simulink model "certasian_traj"  (R2020a)
settings: Solver=VariableStepAuto  StartTime=0.0  StopTime=10.0  RelTol=1e-3
libraries: dsppolyfun x3, simulink x3
settings Model: Creator=UNIST  LastModifiedBy=UNIST

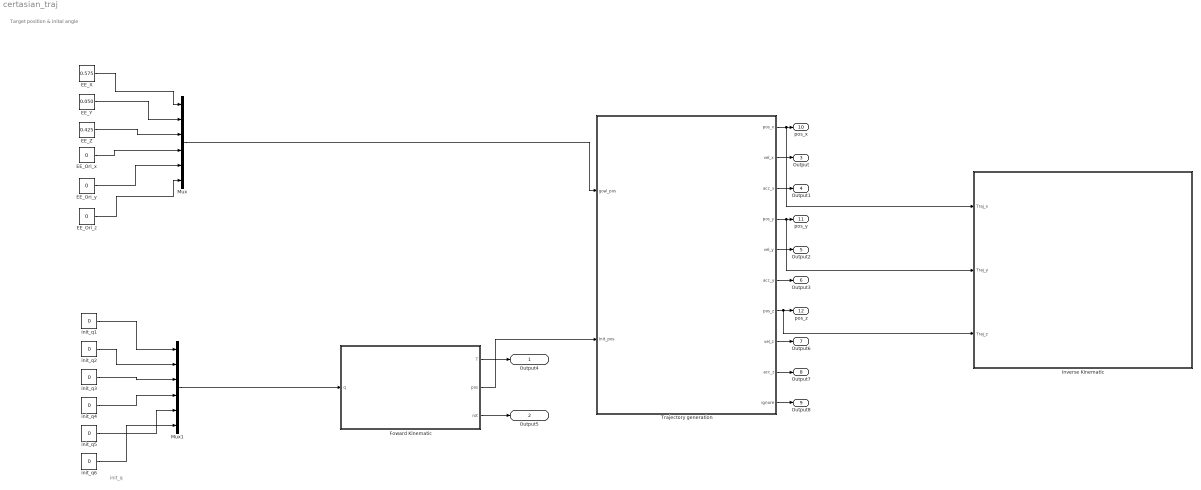
== system certasian_traj ==
  note: Target position & inital angle
  note: init_q
  EE_Ori_x : Constant  Value=0
  EE_Ori_y : Constant  Value=0
  EE_Ori_z : Constant  Value=0
  EE_X : Constant  Value=0.575
  EE_Y : Constant  Value=0.050
  EE_Z : Constant  Value=0.425
  Foward Kinematic : MATLAB Function  TreatAsAtomicUnit=on
  Inverse Kinematic : Subsystem
  Mux : Mux  Inputs=6
  Mux1 : Mux  Inputs=6
  Trajectory generation : Subsystem
  init_q{1..6} (6 alike) : Constant  Value=0
  Output4 : Outport
  Output5 : Outport  Port=2
  Output : Outport  Port=3
  Output1 : Outport  Port=4
  Output2 : Outport  Port=5
  Output3 : Outport  Port=6
  Output6 : Outport  Port=7
  Output7 : Outport  Port=8
  Output8 : Outport  Port=9
  pos_x : Outport  Port=10
  pos_y : Outport  Port=11
  pos_z : Outport  Port=12
  wires:
  EE_Y/1 -> Mux/2
  EE_Ori_x/1 -> Mux/4
  Mux/1 -> Trajectory generation/1(goal_pos)
  init_q6/1 -> Mux1/6
  init_q3/1 -> Mux1/3
  init_q5/1 -> Mux1/5
  EE_Ori_y/1 -> Mux/5
  EE_X/1 -> Mux/1
  init_q1/1 -> Mux1/1
  init_q4/1 -> Mux1/4
  EE_Ori_z/1 -> Mux/6
  init_q2/1 -> Mux1/2
  EE_Z/1 -> Mux/3
  Mux1/1 -> Foward Kinematic/1(q)
  Foward Kinematic/1(T) -> Output4/1
  Foward Kinematic/3(rot) -> Output5/1
  Trajectory generation/2(vel_x) -> Output/1
  Trajectory generation/3(acc_x) -> Output1/1
  Trajectory generation/5(vel_y) -> Output2/1
  Trajectory generation/6(acc_y) -> Output3/1
  Trajectory generation/8(vel_z) -> Output6/1
  Trajectory generation/9(acc_z) -> Output7/1
  Foward Kinematic/2(pos) -> Trajectory generation/2(Init_pos)
  Trajectory generation/10(ignore) -> Output8/1
  Trajectory generation/1(pos_x) -> pos_x/1, Inverse Kinematic/1(Traj_x)
  Trajectory generation/4(pos_y) -> Inverse Kinematic/2(Traj_y), pos_y/1
  Trajectory generation/7(pos_z) -> Inverse Kinematic/3(Traj_z), pos_z/1

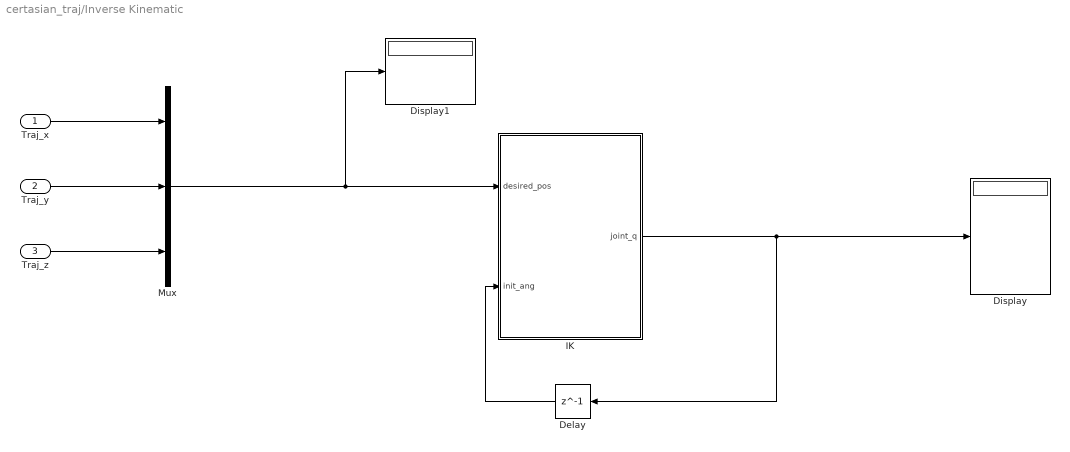
== system certasian_traj/Inverse Kinematic ==
  Traj_x : Inport
  Traj_y : Inport  Port=2
  Traj_z : Inport  Port=3
  Delay : Delay  DelayLength=1
  Display : Display
  Display1 : Display
  IK : MATLAB Function  TreatAsAtomicUnit=on
  Mux : Mux  Inputs=3
  wires:
  Traj_x/1 -> Mux/1
  Traj_y/1 -> Mux/2
  Traj_z/1 -> Mux/3
  Mux/1 -> Display1/1, IK/1(desired_pos)
  IK/1(joint_q) -> Delay/1, Display/1
  Delay/1 -> IK/2(init_ang)

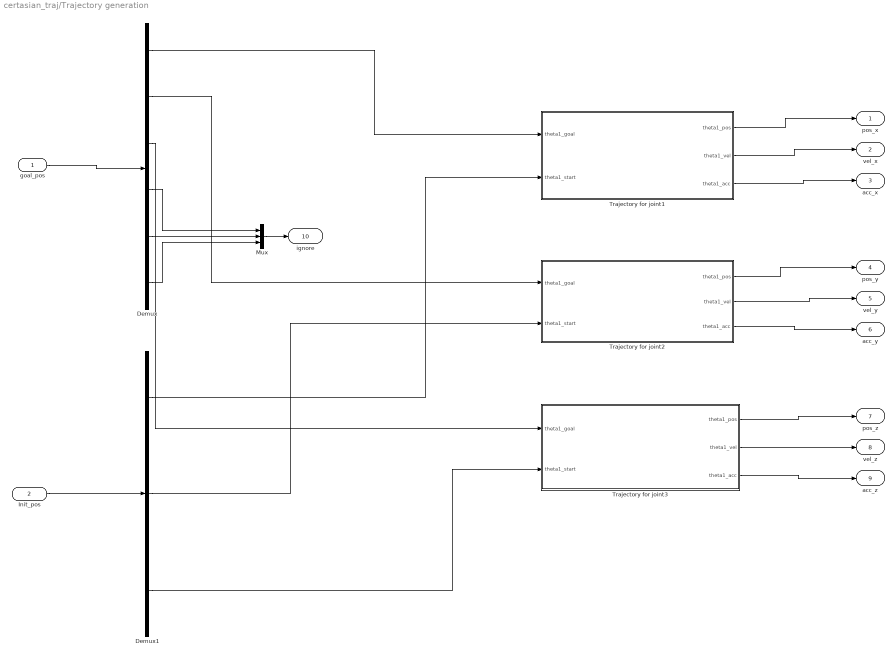
== system certasian_traj/Trajectory generation ==
  goal_pos : Inport
  Init_pos : Inport  Port=2
  Demux : Demux  Outputs=6
  Demux1 : Demux  Outputs=3
  Mux : Mux  Inputs=3
  Trajectory for joint1 : Subsystem
  Trajectory for joint2 : Subsystem
  Trajectory for joint3 : Subsystem
  pos_x : Outport
  vel_x : Outport  Port=2
  acc_x : Outport  Port=3
  pos_y : Outport  Port=4
  vel_y : Outport  Port=5
  acc_y : Outport  Port=6
  pos_z : Outport  Port=7
  vel_z : Outport  Port=8
  acc_z : Outport  Port=9
  ignore : Outport  Port=10
  wires:
  goal_pos/1 -> Demux/1
  Init_pos/1 -> Demux1/1
  Trajectory for joint1/1("theta1_pos ") -> pos_x/1
  Trajectory for joint1/2("theta1_vel ") -> vel_x/1
  Trajectory for joint2/1("theta1_pos ") -> pos_y/1
  Trajectory for joint2/3("theta1_acc ") -> acc_y/1
  Trajectory for joint1/3("theta1_acc ") -> acc_x/1
  Trajectory for joint3/1("theta1_pos ") -> pos_z/1
  Trajectory for joint3/3("theta1_acc ") -> acc_z/1
  Trajectory for joint3/2("theta1_vel ") -> vel_z/1
  Demux/4 -> Mux/1
  Demux/5 -> Mux/2
  Demux/6 -> Mux/3
  Mux/1 -> ignore/1
  Demux/1 -> Trajectory for joint1/1("theta1_goal ")
  Demux1/1 -> Trajectory for joint1/2("theta1_start ")
  Trajectory for joint2/2("theta1_vel ") -> vel_y/1
  Demux/2 -> Trajectory for joint2/1("theta1_goal ")
  Demux1/2 -> Trajectory for joint2/2("theta1_start ")
  Demux/3 -> Trajectory for joint3/1("theta1_goal ")
  Demux1/3 -> Trajectory for joint3/2("theta1_start ")

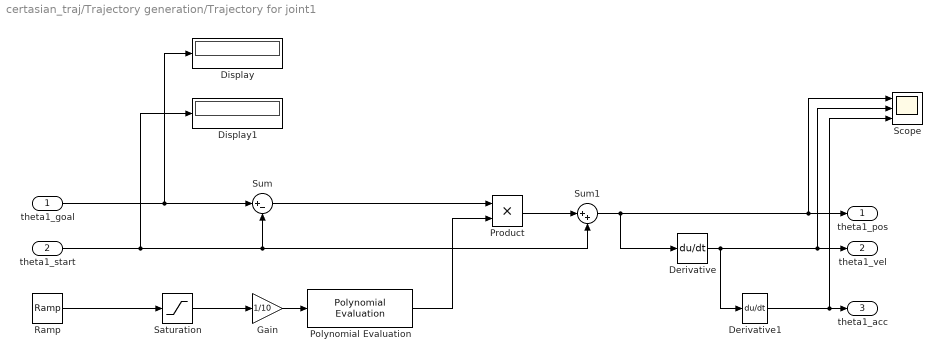
== system certasian_traj/Trajectory generation/Trajectory for joint1 ==
  "theta1_goal " : Inport
  "theta1_start " : Inport  Port=2
  Derivative : Derivative
  Derivative1 : Derivative
  Display : Display
  Display1 : Display
  Gain : Gain  Gain=1/10
  Polynomial Evaluation : dsppolyfun/Polynomial Evaluation  useConstCoeffs=on  constCoeffs=[6 -15 10 0 0 0]
      settings: SourceProductBaseCode=DS
  Product : Product
  Ramp : simulink/Sources/Ramp  slope=1  start=0  InitialOutput=0
  Saturation : Saturate  UpperLimit=10  LowerLimit=-10
  Scope : Scope  NumInputPorts=3
  Sum : Sum  Inputs=|+-
  Sum1 : Sum  Inputs=|++
  "theta1_pos " : Outport  VectorParamsAs1DForOutWhenUnconnected=off
  "theta1_vel " : Outport  Port=2  VectorParamsAs1DForOutWhenUnconnected=off
  "theta1_acc " : Outport  Port=3  VectorParamsAs1DForOutWhenUnconnected=off
  wires:
  "theta1_start "/1 -> Sum1/2, Sum/2, Display1/1
  Sum/1 -> Product/1
  "theta1_goal "/1 -> Display/1, Sum/1
  Sum1/1 -> Derivative/1, Scope/1, "theta1_pos "/1
  Derivative/1 -> Scope/2, "theta1_vel "/1, Derivative1/1
  Gain/1 -> Polynomial Evaluation/1
  Product/1 -> Sum1/1
  Polynomial Evaluation/1 -> Product/2
  Derivative1/1 -> Scope/3, "theta1_acc "/1
  Saturation/1 -> Gain/1
  Ramp/1 -> Saturation/1

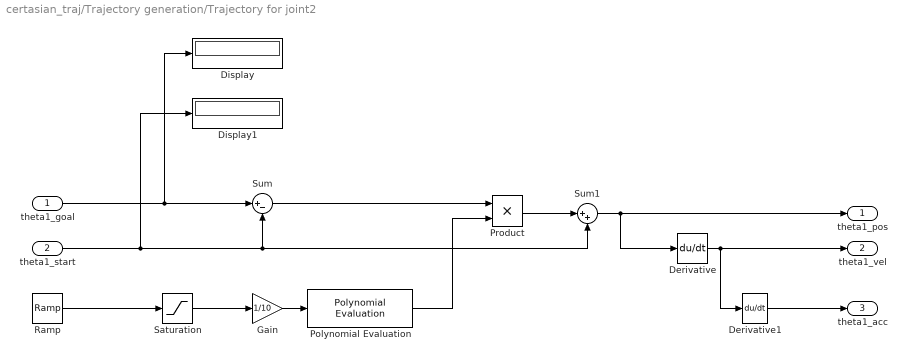
== system certasian_traj/Trajectory generation/Trajectory for joint2 ==
  "theta1_goal " : Inport
  "theta1_start " : Inport  Port=2
  Derivative : Derivative
  Derivative1 : Derivative
  Display : Display
  Display1 : Display
  Gain : Gain  Gain=1/10
  Polynomial Evaluation : dsppolyfun/Polynomial Evaluation  useConstCoeffs=on  constCoeffs=[6 -15 10 0 0 0]
      settings: SourceProductBaseCode=DS
  Product : Product
  Ramp : simulink/Sources/Ramp  slope=1  start=0  InitialOutput=0
  Saturation : Saturate  UpperLimit=10  LowerLimit=-10
  Sum : Sum  Inputs=|+-
  Sum1 : Sum  Inputs=|++
  "theta1_pos " : Outport  VectorParamsAs1DForOutWhenUnconnected=off
  "theta1_vel " : Outport  Port=2  VectorParamsAs1DForOutWhenUnconnected=off
  "theta1_acc " : Outport  Port=3  VectorParamsAs1DForOutWhenUnconnected=off
  wires:
  "theta1_start "/1 -> Sum1/2, Sum/2, Display1/1
  Sum/1 -> Product/1
  "theta1_goal "/1 -> Display/1, Sum/1
  Sum1/1 -> Derivative/1, "theta1_pos "/1
  Derivative/1 -> "theta1_vel "/1, Derivative1/1
  Gain/1 -> Polynomial Evaluation/1
  Product/1 -> Sum1/1
  Polynomial Evaluation/1 -> Product/2
  Derivative1/1 -> "theta1_acc "/1
  Saturation/1 -> Gain/1
  Ramp/1 -> Saturation/1

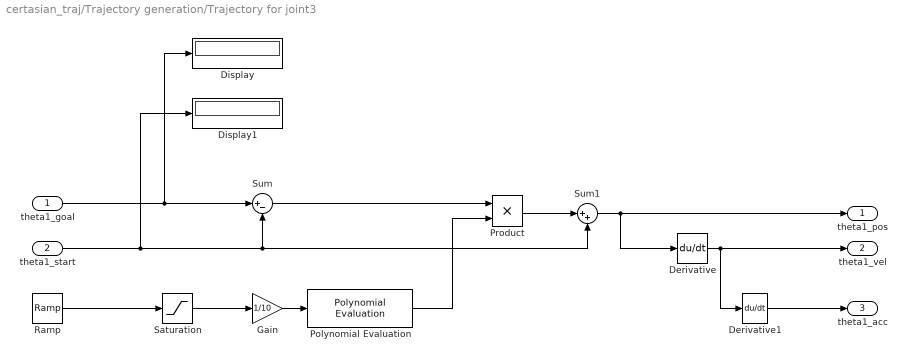
== system certasian_traj/Trajectory generation/Trajectory for joint3 ==
  "theta1_goal " : Inport
  "theta1_start " : Inport  Port=2
  Derivative : Derivative
  Derivative1 : Derivative
  Display : Display
  Display1 : Display
  Gain : Gain  Gain=1/10
  Polynomial Evaluation : dsppolyfun/Polynomial Evaluation  useConstCoeffs=on  constCoeffs=[6 -15 10 0 0 0]
      settings: SourceProductBaseCode=DS
  Product : Product
  Ramp : simulink/Sources/Ramp  slope=1  start=0  InitialOutput=0
  Saturation : Saturate  UpperLimit=10  LowerLimit=-10
  Sum : Sum  Inputs=|+-
  Sum1 : Sum  Inputs=|++
  "theta1_pos " : Outport  VectorParamsAs1DForOutWhenUnconnected=off
  "theta1_vel " : Outport  Port=2  VectorParamsAs1DForOutWhenUnconnected=off
  "theta1_acc " : Outport  Port=3  VectorParamsAs1DForOutWhenUnconnected=off
  wires:
  "theta1_start "/1 -> Sum1/2, Sum/2, Display1/1
  Sum/1 -> Product/1
  "theta1_goal "/1 -> Display/1, Sum/1
  Sum1/1 -> Derivative/1, "theta1_pos "/1
  Derivative/1 -> "theta1_vel "/1, Derivative1/1
  Gain/1 -> Polynomial Evaluation/1
  Product/1 -> Sum1/1
  Polynomial Evaluation/1 -> Product/2
  Derivative1/1 -> "theta1_acc "/1
  Saturation/1 -> Gain/1
  Ramp/1 -> Saturation/1

== matlab function certasian_traj/Foward Kinematic ==
  data: q input; T output; pos output; rot output
function [T,pos,rot] = FK(q)

theta1=q(1);  d1=0;   a1=0.050;  alpha1=-90; %parameter link1
theta2=q(2);  d2=0.050;   a2=0.425;  alpha2=0; %parameter link2
theta3=q(3);  d3=0;  a3=0;  alpha3=90; %parameter link3
theta4=q(4);  d4=0.425;   a4=0;  alpha4=-90; %parameter link4
theta5=q(5);  d5=0; a5=0;  alpha5=90; %parameter link5
theta6=q(6);  d6=0.100; a6=0;  alpha6=0; %parameter link6
offset2 = -90;
offset3 = 90;
T01=[cosd(theta1) -cosd(alpha1)*sind(theta1) sind(alpha1)*sind(theta1) a1*cosd(theta1);
    sind(theta1) cosd(alpha1)*cosd(theta1)  -sind(alpha1)*cosd(theta1) a1*sind(theta1);
    0,sind(alpha1),cosd(alpha1),d1;
    0,0,0,1];
T12=[cosd(theta2+offset2) -cosd(alpha2)*sind(theta2+offset2) sind(alpha2)*sind(theta2+offset2) a2*cosd(theta2+offset2);
    sind(theta2+offset2) cosd(alpha2)*cosd(theta2+offset2)  -sind(alpha2)*cosd(theta2+offset2) a2*sind(theta2+offset2);
    0,sind(alpha2),cosd(alpha2),d2;
    0,0,0,1];
T23=[cosd(theta3+offset3) -cosd(alpha3)*sind(theta3+offset3) sind(alpha3)*sind(theta3+offset3) a3*cosd(theta3+offset3);
    sind(theta3+offset3) cosd(alpha3)*cosd(theta3+offset3)  -sind(alpha3)*cosd(theta3+offset3) a3*sind(theta3+offset3);
    0,sind(alpha3),cosd(alpha3),d3;
    0,0,0,1];
T34=[cosd(theta4) -cosd(alpha4)*sind(theta4) sind(alpha4)*sind(theta4) a4*cosd(theta4);
     sind(theta4) cosd(alpha4)*cosd(theta4)  -sind(alpha4)*cosd(theta4) a4*sind(theta4);
     0,sind(alpha4),cosd(alpha4),d4;
     0,0,0,1];
T45=[cosd(theta5) -cosd(alpha5)*sind(theta5) sind(alpha5)*sind(theta5) a5*cosd(theta5);
     sind(theta5) cosd(alpha5)*cosd(theta5)  -sind(alpha5)*cosd(theta5) a5*sind(theta5);
     0,sind(alpha5),cosd(alpha5),d5;
     0,0,0,1];
T56=[cosd(theta6) -cosd(alpha6)*sind(theta6) sind(alpha6)*sind(theta6) a6*cosd(theta6);
     sind(theta6) cosd(alpha6)*cosd(theta6)  -sind(alpha6)*cosd(theta6) a6*sind(theta6);
     0,sind(alpha6),cosd(alpha6),d6;
     0,0,0,1];
T01;
T02 = T01*T12;
T03 = T01*T12*T23;
T04 = T01*T12*T23*T34;
T05 = T01*T12*T23*T34*T45;
T06 = T01*T12*T23*T34*T45*T56;
P6=T06(1:3,4);
R = [T06(1:3,1) T06(1:3,2) T06(1:3,3)]; 
T = T06;
pos = P6;
rot = R;

== matlab function certasian_traj/Inverse Kinematic/IK ==
  data: desired_pos input; joint_q output; init_ang input
function joint_q = IK(desired_pos, init_ang)

theta1=init_ang(1);  d1=0;   a1=0.050;  alpha1=-90; %parameter link1
theta2=init_ang(2);  d2=0.050;   a2=0.425;  alpha2=0; %parameter link2
theta3=init_ang(3);  d3=0;  a3=0;  alpha3=90; %parameter link3
theta4=init_ang(4);  d4=0.425;   a4=0;  alpha4=-90; %parameter link4
theta5=init_ang(5);  d5=0; a5=0;  alpha5=90; %parameter link5
theta6=init_ang(6);  d6=0.100; a6=0;  alpha6=0; %parameter link6

offset2 = -90;
offset3 = 90;

T01=[cosd(theta1) -cosd(alpha1)*sind(theta1) sind(alpha1)*sind(theta1) a1*cosd(theta1);
sind(theta1) cosd(alpha1)*cosd(theta1)  -sind(alpha1)*cosd(theta1) a1*sind(theta1);
0,sind(alpha1),cosd(alpha1),d1;
0,0,0,1];
T12=[cosd(theta2+offset2) -cosd(alpha2)*sind(theta2+offset2) sind(alpha2)*sind(theta2+offset2) a2*cosd(theta2+offset2);
sind(theta2+offset2) cosd(alpha2)*cosd(theta2+offset2)  -sind(alpha2)*cosd(theta2+offset2) a2*sind(theta2+offset2);
0,sind(alpha2),cosd(alpha2),d2;
0,0,0,1];
T23=[cosd(theta3+offset3) -cosd(alpha3)*sind(theta3+offset3) sind(alpha3)*sind(theta3+offset3) a3*cosd(theta3+offset3);
sind(theta3+offset3) cosd(alpha3)*cosd(theta3+offset3)  -sind(alpha3)*cosd(theta3+offset3) a3*sind(theta3+offset3);
0,sind(alpha3),cosd(alpha3),d3;
0,0,0,1];
T34=[cosd(theta4) -cosd(alpha4)*sind(theta4) sind(alpha4)*sind(theta4) a4*cosd(theta4);
 sind(theta4) cosd(alpha4)*cosd(theta4)  -sind(alpha4)*cosd(theta4) a4*sind(theta4);
 0,sind(alpha4),cosd(alpha4),d4;
 0,0,0,1];
T45=[cosd(theta5) -cosd(alpha5)*sind(theta5) sind(alpha5)*sind(theta5) a5*cosd(theta5);
 sind(theta5) cosd(alpha5)*cosd(theta5)  -sind(alpha5)*cosd(theta5) a5*sind(theta5);
 0,sind(alpha5),cosd(alpha5),d5;
 0,0,0,1];
T56=[cosd(theta6) -cosd(alpha6)*sind(theta6) sind(alpha6)*sind(theta6) a6*cosd(theta6);
 sind(theta6) cosd(alpha6)*cosd(theta6)  -sind(alpha6)*cosd(theta6) a6*sind(theta6);
 0,sind(alpha6),cosd(alpha6),d6;
 0,0,0,1];
T01;
T02 = T01*T12;
T03 = T01*T12*T23;
T04 = T01*T12*T23*T34;
T05 = T01*T12*T23*T34*T45;
T06 = T01*T12*T23*T34*T45*T56;
P6=T06(1:3,4);
iteration = 0;
b = 0 ;
deltatheta1=0;deltatheta2=0; deltatheta3=0; %theta1,2,3 velocity
deltatheta4=0;deltatheta5=0; deltatheta6=0; %theta4,5,6 velocity
    while b == 0
        if theta1 >180
            theta1 = -180 + theta1;
        elseif theta1 <-180
            theta1 = -theta1;
        end
        if theta2+offset2 >147.5
            theta2 = -147.5 + theta2;
        elseif theta2+offset2 <-130
            theta2 = -theta2;
        end
        if theta3 >145
            theta3 = -145 + theta3;
        elseif theta3 <-145
            theta3 = -theta3;
        end
        if theta4 >270
            theta4 = -270 + theta4;
        elseif theta4 <-270
            theta4 = -theta4;
        end
        if theta5 >140
            theta5 = -140 + theta5;
        elseif theta5 <-115
            theta5 = -theta5;
        end
        if theta6 >270
            theta6 = -270 + theta6;
        elseif theta6 <-270
            theta6 = -theta6;
        end
    %     result = [theta1 theta2 theta3 theta4 theta5 theta6];
    %     disp("result"); disp(result);
        theta1=theta1+deltatheta1/2;
        theta2=theta2+deltatheta2/2;
        theta3=theta3+deltatheta3/2;
        theta4=theta4+deltatheta4/2;
        theta5=theta5+deltatheta5/2;
        theta6=theta6+deltatheta6/2;
        theta = [theta1 theta2 theta3 theta4 theta5 theta6];
        if(iteration > 100000)
            % avoid too many calculation
            b=1;
            iteration = 0;
        end
        T01=[cosd(theta1) -cosd(alpha1)*sind(theta1) sind(alpha1)*sind(theta1) a1*cosd(theta1);
            sind(theta1) cosd(alpha1)*cosd(theta1)  -sind(alpha1)*cosd(theta1) a1*sind(theta1);
            0,sind(alpha1),cosd(alpha1),d1;
            0,0,0,1];
        T12=[cosd(theta2+offset2) -cosd(alpha2)*sind(theta2+offset2) sind(alpha2)*sind(theta2+offset2) a2*cosd(theta2+offset2);
            sind(theta2+offset2) cosd(alpha2)*cosd(theta2+offset2)  -sind(alpha2)*cosd(theta2+offset2) a2*sind(theta2+offset2);
            0,sind(alpha2),cosd(alpha2),d2;
            0,0,0,1];
        T23=[cosd(theta3+offset3) -cosd(alpha3)*sind(theta3+offset3) sind(alpha3)*sind(theta3+offset3) a3*cosd(theta3+offset3);
            sind(theta3+offset3) cosd(alpha3)*cosd(theta3+offset3)  -sind(alpha3)*cosd(theta3+offset3) a3*sind(theta3+offset3);
            0,sind(alpha3),cosd(alpha3),d3;
            0,0,0,1];
        T34=[cosd(theta4) -cosd(alpha4)*sind(theta4) sind(alpha4)*sind(theta4) a4*cosd(theta4);
             sind(theta4) cosd(alpha4)*cosd(theta4)  -sind(alpha4)*cosd(theta4) a4*sind(theta4);
             0,sind(alpha4),cosd(alpha4),d4;
             0,0,0,1];
        T45=[cosd(theta5) -cosd(alpha5)*sind(theta5) sind(alpha5)*sind(theta5) a5*cosd(theta5);
             sind(theta5) cosd(alpha5)*cosd(theta5)  -sind(alpha5)*cosd(theta5) a5*sind(theta5);
             0,sind(alpha5),cosd(alpha5),d5;
             0,0,0,1];
        T56=[cosd(theta6) -cosd(alpha6)*sind(theta6) sind(alpha6)*sind(theta6) a6*cosd(theta6);
             sind(theta6) cosd(alpha6)*cosd(theta6)  -sind(alpha6)*cosd(theta6) a6*sind(theta6);
             0,sind(alpha6),cosd(alpha6),d6;
             0,0,0,1];
        T01;
        T02 = T01*T12;
        T03 = T01*T12*T23;
        T04 = T01*T12*T23*T34;
        T05 = T01*T12*T23*T34*T45;
        T06 = T01*T12*T23*T34*T45*T56;

        P0=[0 0 0]';
        P1=T01(1:3,4);
        P2=T02(1:3,4);
        P3=T03(1:3,4);
        P4=T04(1:3,4);
        P5=T05(1:3,4);
        P6=T06(1:3,4);
        %%%%%%%%%%%%%%%%%%%%%%%
        Z0  = [0;0;1];
        Jv1 = cross(Z0,(P6-P0));

        Z1  = T01(1:3,3);
        Jv2 = cross(Z1,(P6-P1));

        Z2  = T02(1:3,3);
        Jv3 = cross(Z2,(P6-P2));

        Z3  = T03(1:3,3);
        Jv4 = cross(Z3,(P6-P3));

        Z4  = T04(1:3,3);
        Jv5 = cross(Z4,(P6-P4));

        Z5  = T05(1:3,3);
        Jv6 = cross(Z5,(P6-P5));
        Jv=[Jv1 Jv2 Jv3 Jv4 Jv5 Jv6];
            %Z0   Z1  Z2  Z3  Z4  Z5]

        Xinit=P6(1,1); 
        Yinit=P6(2,1);
        Zinit = P6(3,1);

        Xspeed=desired_pos(1)-Xinit;
        Yspeed=desired_pos(2)-Yinit;
        Zspeed=desired_pos(3)-Zinit;

        thetadot=pinv(Jv)*[Xspeed;Yspeed;Zspeed];
        error_x = Xspeed;
        error_y = Yspeed;
        error_z = Zspeed;

        if abs(error_x)<=0.001 && abs(error_y)<=0.001 && abs(error_z)<=0.001 %&& abs(error_r)<=0.5 && abs(error_p)<=0.5 && abs(error_yaw)<=0.5
            disp("here?")
            End_EE = T06;
            b=1;
        end
        theta1dot=thetadot(1,1);
        theta2dot=thetadot(2,1);
        theta3dot=thetadot(3,1);
        theta4dot=thetadot(4,1);
        theta5dot=thetadot(5,1);
        theta6dot=thetadot(6,1);

        deltatheta1=rad2deg(theta1dot);
        deltatheta2=rad2deg(theta2dot);
        deltatheta3=rad2deg(theta3dot);
        deltatheta4=rad2deg(theta4dot);
        deltatheta5=rad2deg(theta5dot);
        deltatheta6=rad2deg(theta6dot);
        iteration = iteration +1;
    end
theta_final = [theta1 theta2 theta3 theta4 theta5 theta6];
joint_q = theta_final;
end
